simulink model "polinomial_ord3"  (R2018a)
settings: Solver=FixedStepAuto  StartTime=0.0  StopTime=25  FixedStep=0.01  RelTol=1e-3
undefined symbols (not defined in the file): C, F, G, P1
libraries: arduino_io_lib x5
settings Model: Creator=Mauricio  LastModifiedBy=Mauricio

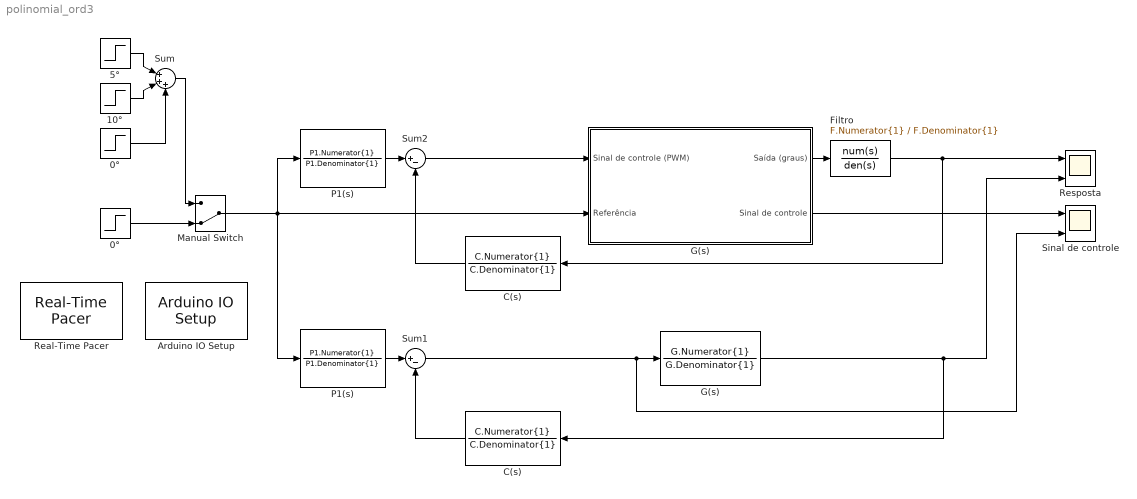
== system polinomial_ord3 ==
  0° : Step  Time=0  After=0  SampleTime=0.05
  "0° " : Step  Time=15  After=-9  SampleTime=0.05
  10° : Step  Time=10  After=3  SampleTime=0.05
  5° : Step  Time=5  After=6  SampleTime=0.05
  Arduino IO Setup : arduino_io_lib/Arduino IO Setup  Priority=3  arduinoVar=Temporary arduino variable: Arduino1  workspaceVarName=a  comPort=COM4
  C(s) : TransferFcn  Numerator=C.Numerator{1}  Denominator=C.Denominator{1}
  "C(s) " : TransferFcn  Numerator=C.Numerator{1}  Denominator=C.Denominator{1}
  Filtro : TransferFcn  Numerator=F.Numerator{1}  Denominator=F.Denominator{1}
  G(s) : TransferFcn  Numerator=G.Numerator{1}  Denominator=G.Denominator{1}
  "G(s) " : Subsystem
  Manual Switch : ManualSwitch  CurrentSetting=0
  P1(s) : TransferFcn  Numerator=P1.Numerator{1}  Denominator=P1.Denominator{1}
  "P1(s) " : TransferFcn  Numerator=P1.Numerator{1}  Denominator=P1.Denominator{1}
  Real-Time Pacer : arduino_io_lib/Real-Time Pacer  simTimePerRealTime=1
  Resposta : Scope  NumInputPorts=2
  Sinal de controle : Scope  NumInputPorts=2
  Sum : Sum  Inputs=|+++
  Sum1 : Sum  Inputs=|+-
  Sum2 : Sum  Inputs=|+-
  wires:
  "G(s) "/1(Saída (graus)) -> Filtro/1
  G(s)/1 -> Resposta/2, "C(s) "/1
  "G(s) "/2(Sinal de controle) -> Sinal de controle/1
  5°/1 -> Sum/1
  0°/1 -> Manual Switch/2
  Sum/1 -> Manual Switch/1
  Filtro/1 -> C(s)/1, Resposta/1
  Sum2/1 -> "G(s) "/1(Sinal de controle (PWM))
  10°/1 -> Sum/2
  "0° "/1 -> Sum/3
  Manual Switch/1 -> "P1(s) "/1, "G(s) "/2(Referência), P1(s)/1
  "P1(s) "/1 -> Sum1/1
  P1(s)/1 -> Sum2/1
  Sum1/1 -> Sinal de controle/2, G(s)/1
  C(s)/1 -> Sum2/2
  "C(s) "/1 -> Sum1/2

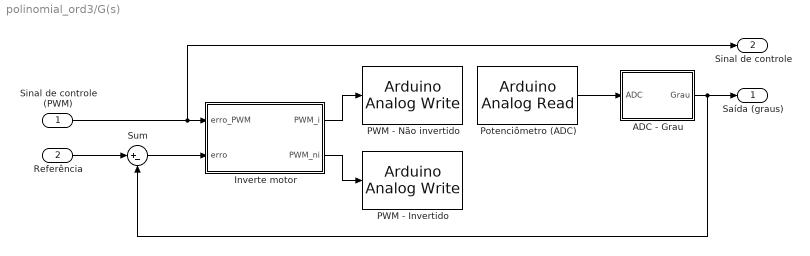
== system polinomial_ord3/G(s)  ==
  Sinal de controle (PWM) : Inport
  Referência : Inport  Port=2
  ADC - Grau : MATLAB Function  TreatAsAtomicUnit=on
  Inverte motor : MATLAB Function  TreatAsAtomicUnit=on
  PWM - Invertido : arduino_io_lib/Arduino Analog Write  arduinoVar=Temporary arduino variable: Arduino1  arduinoPin=6  T=0.05
  PWM - Não invertido : arduino_io_lib/Arduino Analog Write  arduinoVar=Temporary arduino variable: Arduino1  arduinoPin=5  T=0.05
  Potenciômetro (ADC) : arduino_io_lib/Arduino Analog Read  arduinoVar=Temporary arduino variable: Arduino1  arduinoPin=2  T=0.01
  Sum : Sum  Inputs=|+-
  Saída (graus) : Outport
  Sinal de controle : Outport  Port=2
  wires:
  Potenciômetro (ADC)/1 -> ADC - Grau/1(ADC)
  Inverte motor/2(PWM_ni) -> PWM - Invertido/1
  Inverte motor/1(PWM_i) -> PWM - Não invertido/1
  ADC - Grau/1(Grau) -> Sum/2, Saída (graus)/1
  Sum/1 -> Inverte motor/2(erro)
  Referência/1 -> Sum/1
  Sinal de controle (PWM)/1 -> Sinal de controle/1, Inverte motor/1(erro_PWM)

== matlab function polinomial_ord3/G(s) /ADC - Grau ==
  data: ADC input; Grau output
function Grau = fcn(ADC)
Grau = -0.17413322126497163269594452616096*ADC + 136.2690584156335364572389157386;

== matlab function polinomial_ord3/G(s) /Inverte motor ==
  data: PWM_i output; PWM_ni output; erro_PWM input; erro input
function [PWM_i, PWM_ni] = fcn(erro_PWM, erro)
%erro_PWM representa o sinal de controle, dado em PWM
%erro representa a diferenca entre o sinal de saida e a referencia

dead_zone = 45; %zona morta do motor CC em torno do 0°.
erro_permissivel = 0.75; %erro aceitavel para a saida do sistema

%Confere se a saida esta dentro do erro aceitavel, ja que nao existe
%integrador no controlador
if(abs(erro) <= erro_permissivel)
    erro_PWM = 0;
end

%DESLIGADO
if(erro_PWM == 0)
    PWM_ni = 0;
    PWM_i = 0;
%REVERSO
elseif(erro_PWM>0)
    erro_PWM = erro_PWM + dead_zone; 
    PWM_i = erro_PWM;
    PWM_ni = 0;
%DIRETO
else
    erro_PWM = erro_PWM - dead_zone;
    PWM_ni = abs(erro_PWM);
    PWM_i = 0;
end
